simulink model "platoon111311fixpoint"  (Simulink 7.9)
settings: Solver=ode45  StartTime=0.0  StopTime=10.0  RelTol=1e-3
settings Model: Creator=Norman  LastModifiedBy=Norman

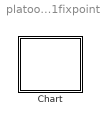
== system platoon111311fixpoint ==
  Chart : Stateflow chart  TreatAsAtomicUnit=on

== stateflow chart Chart ==
  state a" ==     b &
    b" ==    -c + u&
    c" ==     1.6050a    +4.8680b   -3.5754c   -0.8198d   + 0.4270e   -0.0450f   -0.1942g   + 0.3626h   -0.0946i &
    d" ==     e &
    e "==     c -f &
    f" ==      0.8718a    +3.8140b  -0.0754c   + 1.1936d   + 3.6258e   -3.2396f   -0.5950g   + 0.1294h   -0.0796i &
    g" ==     h &
    h"==      f -i &
    i"==       0.7132a   + 3.5730b   -0.0964c   + 0.8472d    +3.2568e   -0.0876f   + 1.2726g   + 3.0720h   -3.1356i
  state a" ==  b &
    b" ==       -c+u &
    c" ==        1.6050a    +4.8680b   -3.5754c      &
    d" ==       e &
    e" ==      c -f&
    f" ==       1.1936d  +  3.6258e   -3.2396 f      &
    g" ==   h &
    h" ==       f      - i&
    i" ==   0.7132a  +3.5730b  -0.0964c  +  0.8472d +  3.2568e  -0.0876 f  + 1.2726g   + 3.0720 h  -3.1356i
  (default) -> a" ==     b &
  a" ==     b & -> a" ==  b & : fixpoint
  a" ==  b & -> a" ==     b & : fixpoint
